simulink model "OpenLoopLinearModel"  (R2016a)
settings: Solver=ode15s  StartTime=0.0  StopTime=70  MaxStep=1e-3  MinStep=1e-5  RelTol=1e-3
values from neighbouring files (symbols this model uses):
  A = 'elevation'    [importdata.m]    (also in setup_lab_heli_3d.m = zeros(6,6))
  B = zeros(6,2)    [setup_lab_heli_3d.m]
  C = 'pitch'    [importdata.m]    (also in setup_lab_heli_3d.m = eye(6))
  D = 'travel'    [importdata.m]    (also in setup_lab_heli_3d.m = zeros(6,2))
  K_AMP = 3    [setup_lab_heli_3d.m]
  VMAX_AMP = 24    [setup_lab_heli_3d.m]
  VMAX_DAC = 10    [setup_lab_heli_3d.m]
libraries: simulink_extras x1
settings Model: Creator=ap4614  LastModifiedBy=jcg216
settings DataIOCC: SaveFormat=Array
settings HardwareCC: ProdBitPerPointer=32  ProdLargestAtomicFloat=None  ProdIntDivRoundTo=Undefined  ProdEndianess=Unspecified  ProdWordSize=32  ProdHWDeviceType=32-bit Generic
settings ModelReferenceCC: PropagateSignalLabelsOutOfModel=off
settings ConfigComp: CovModelRefEnable=Off

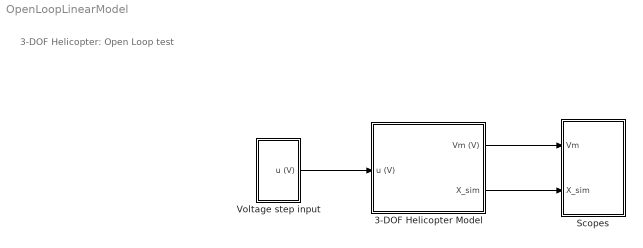
== system OpenLoopLinearModel ==
  note: 3-DOF Helicopter: Open Loop test
  3-DOF Helicopter Model : Subsystem
  Scopes : Subsystem
  Voltage step input : Subsystem
  wires:
  Voltage step input/1(u (V)) -> 3-DOF Helicopter Model/1(u (V))
  3-DOF Helicopter Model/2(X_sim) -> Scopes/2(X_sim)
  3-DOF Helicopter Model/1(Vm (V)) -> Scopes/1(Vm)

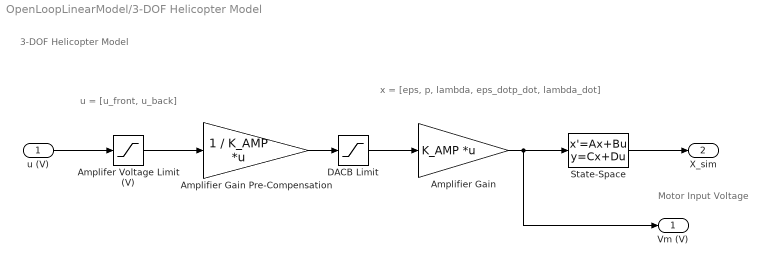
== system OpenLoopLinearModel/3-DOF Helicopter Model ==
  note: x = [eps, p, lambda, eps_dotp_dot, lambda_dot]
  note: u = [u_front, u_back]
  note: Motor Input Voltage
  note: 3-DOF Helicopter Model
  u (V) : Inport
  Amplifer Voltage Limit (V) : Saturate  UpperLimit=VMAX_AMP  LowerLimit=-VMAX_AMP
  Amplifier Gain : Gain  Gain=K_AMP  Multiplication=Matrix(K*u)  SaturateOnIntegerOverflow=on  OutDataTypeStr=Inherit: Same as input  ParamDataTypeStr=Inherit: Same as input
  Amplifier Gain Pre-Compensation : Gain  Gain=1 / K_AMP  Multiplication=Matrix(K*u)  SaturateOnIntegerOverflow=on  OutDataTypeStr=Inherit: Same as input  ParamDataTypeStr=Inherit: Same as input
  DACB Limit : Saturate  UpperLimit=VMAX_DAC  LowerLimit=-VMAX_DAC
  State-Space : StateSpace  A=A  B=B  C=C  D=D  X0=0
  Vm (V) : Outport
  X_sim : Outport  Port=2
  wires:
  u (V)/1 -> Amplifer Voltage Limit (V)/1
  Amplifier Gain/1 -> State-Space/1, Vm (V)/1
  Amplifer Voltage Limit (V)/1 -> Amplifier Gain Pre-Compensation/1
  Amplifier Gain Pre-Compensation/1 -> DACB Limit/1
  DACB Limit/1 -> Amplifier Gain/1
  State-Space/1 -> X_sim/1

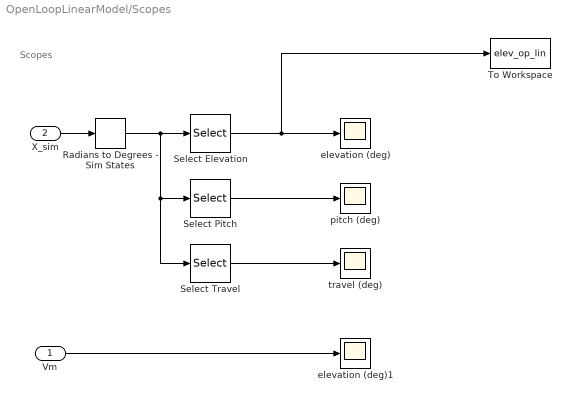
== system OpenLoopLinearModel/Scopes ==
  note: Scopes
  Vm : Inport
  X_sim : Inport  Port=2
  Radians to Degrees - Sim States : simulink_extras/Transformations/Radians to Degrees
  Select Elevation : Selector  InputPortWidth=6  IndexOptions=Index vector (dialog)  Indices=1  OutputSizes=1
  Select Pitch : Selector  InputPortWidth=6  IndexOptions=Index vector (dialog)  Indices=2  OutputSizes=1
  Select Travel : Selector  InputPortWidth=6  IndexOptions=Index vector (dialog)  Indices=3  OutputSizes=1
  To Workspace : ToWorkspace  VariableName=elev_op_lin  SampleTime=-1
  elevation (deg) : Scope
  elevation (deg)1 : Scope
  pitch (deg) : Scope
  travel (deg) : Scope
  wires:
  X_sim/1 -> Radians to Degrees - Sim States/1
  Select Elevation/1 -> To Workspace/1, elevation (deg)/1
  Vm/1 -> elevation (deg)1/1
  Radians to Degrees - Sim States/1 -> Select Elevation/1, Select Pitch/1, Select Travel/1
  Select Travel/1 -> travel (deg)/1
  Select Pitch/1 -> pitch (deg)/1

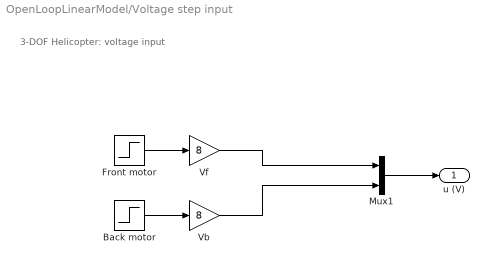
== system OpenLoopLinearModel/Voltage step input ==
  note: 3-DOF Helicopter: voltage input
  Back motor : Step  SampleTime=0
  Front motor : Step  SampleTime=0
  Mux1 : Mux  Inputs=2
  "Vb " : Gain  Gain=8
  Vf : Gain  Gain=8
  u (V) : Outport
  wires:
  Mux1/1 -> u (V)/1
  Front motor/1 -> Vf/1
  Back motor/1 -> "Vb "/1
  Vf/1 -> Mux1/1
  "Vb "/1 -> Mux1/2
